simulink model "GPCA_Logging_tmp"  (Simulink 8.4)
settings: Solver=ode45  StartTime=0.0  StopTime=10.0  RelTol=1e-3
settings Model: Creator=bourbouh  LastModifiedBy=hbourbou  CovSFcnEnable=on
settings DataIOCC: LimitDataPoints=off  SaveFormat=StructureWithTime  SignalLoggingSaveFormat=Dataset
settings OptimizationCC: ExpressionDepthLimit=128
settings DebuggingCC: UnderspecifiedInitializationDetection=Simplified  MergeDetectMultiDrivingBlocksExec=error  SolverPrmCheckMsg=none  FcnCallInpInsideContextMsg=EnableAllAsError  FrameProcessingCompatibilityMsg=error  StateNameClashWarn=none
settings HardwareCC: ProdBitPerPointer=64  ProdLargestAtomicFloat=Float  ProdIntDivRoundTo=Zero  ProdEndianess=LittleEndian  ProdHWDeviceType=Specified
settings ModelReferenceCC: PropagateSignalLabelsOutOfModel=on
settings GRTTargetCC: CombineOutputUpdateFcns=on  GRTInterface=off

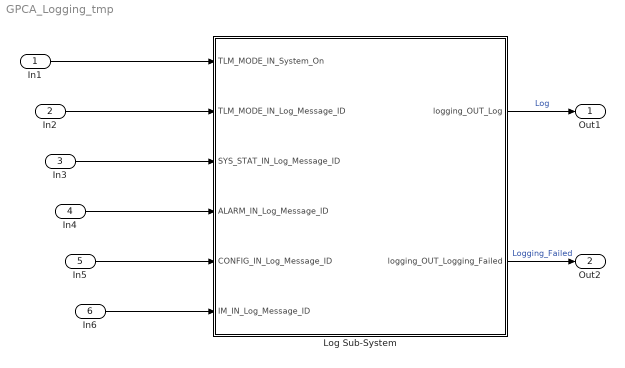
== system GPCA_Logging_tmp ==
  In1 : Inport
  In2 : Inport  Port=2
  In3 : Inport  Port=3
  In4 : Inport  Port=4
  In5 : Inport  Port=5
  In6 : Inport  Port=6
  Log Sub-System : Stateflow chart  TreatAsAtomicUnit=on
      settings: PermitHierarchicalResolution=ParametersOnly
  Out1 : Outport
  Out2 : Outport  Port=2
  wires:
  In1/1 -> Log Sub-System/1(TLM_MODE_IN_System_On)
  In2/1 -> Log Sub-System/2(TLM_MODE_IN_Log_Message_ID)
  In3/1 -> Log Sub-System/3(SYS_STAT_IN_Log_Message_ID)
  In4/1 -> Log Sub-System/4(ALARM_IN_Log_Message_ID)
  In5/1 -> Log Sub-System/5(CONFIG_IN_Log_Message_ID)
  In6/1 -> Log Sub-System/6(IM_IN_Log_Message_ID)
  Log Sub-System/1(logging_OUT_Log) -> Out1/1  "Log"
  Log Sub-System/2(logging_OUT_Logging_Failed) -> Out2/1  "Logging_Failed"

== stateflow chart Log Sub-System ==
  state NOT_ON
    entry: logging_OUT_Log=0;
    during : logging_OUT_Log=0;
    exit: logging_OUT_Log=0;
  state LOG
    entry: logging_OUT_Logging_Failed=0;
    logging_OUT_Log= writeLog(TLM_MODE_IN_Log_Message_ID, SYS_STAT_IN_Log_Message_ID, ALARM_IN_Log_Message_ID, CONFIG_IN_Log_Message_ID, IM_IN_Log_Message_ID)
    during: logging_OUT_Logging_Failed=0;
    logging_OUT_Log= writeLog(TLM_MODE_IN_Log_Message_ID, SYS_STAT_IN_Log_Message_ID, ALARM_IN_Log_Message_ID, CONFIG_IN_Log_Message_ID, IM_IN_Log_Message_ID)
    exit: logging_OUT_Logging_Failed=0;
    logging_OUT_Log= writeLog(TLM_MODE_IN_Log_Message_ID, SYS_STAT_IN_Log_Message_ID, ALARM_IN_Log_Message_ID, CONFIG_IN_Log_Message_ID, IM_IN_Log_Message_ID)
  note: Functionality shall be added later. For now its just a place holder
  state logging_OUT_Log= writeLog(TLM_MODE_IN_Log_Message_ID, SYS_STAT_IN_Log_Message_ID, ALARM_IN_Log_Message_ID, CONFIG_IN_Log_Message_ID, IM_IN_Log_Message_ID) [function]
    (default) -> (junction 13) : {logging_OUT_Log=0;}
    (junction 13) -> (junction 14) : [(TLM_MODE_IN_Log_Message_ID > 0) || (SYS_STAT_IN_Log_Message_ID > 0)  || (ALARM_IN_Log_Message_ID > 0)  ||  (CONFIG_IN_Log_Message_ID > 0)  || (IM_IN_Log_Message_ID > 0)]{logging_OUT_Log=1;}
  (default) -> NOT_ON [order 2]
  (default) -> LOG [order 1] : [TLM_MODE_IN_System_On]
  NOT_ON -> LOG : [TLM_MODE_IN_System_On]
  LOG -> NOT_ON : [!TLM_MODE_IN_System_On]
  data: logging_OUT_Log function_output uint8; TLM_MODE_IN_Log_Message_ID function_input uint8; SYS_STAT_IN_Log_Message_ID function_input uint8; ALARM_IN_Log_Message_ID function_input uint8; CONFIG_IN_Log_Message_ID function_input uint8; IM_IN_Log_Message_ID function_input uint8; TLM_MODE_IN_System_On input boolean; TLM_MODE_IN_Log_Message_ID input uint8; SYS_STAT_IN_Log_Message_ID input uint8; ALARM_IN_Log_Message_ID input uint8; CONFIG_IN_Log_Message_ID input uint8; logging_OUT_Log output uint8; logging_OUT_Logging_Failed output boolean; IM_IN_Log_Message_ID input uint8
